simulink model "wavelet_transmux"  (R2018a)
settings: Solver=FixedStepDiscrete  StartTime=0.0  StopTime=inf  RelTol=1e-3
libraries: dspmlti4 x2, dspsrcs4 x1
settings Model: Creator=Kaustubh  LastModifiedBy=Kaustubh
settings SolverCC: AutoInsertRateTranBlk=on
settings DataIOCC: LimitDataPoints=on  SaveOutput=off  SignalLogging=off  SaveTime=off
settings OptimizationCC: LifeSpan=inf  SimCompilerOptimization=on
settings DebuggingCC: AlgebraicLoopMsg=error  SingleTaskRateTransMsg=error  AllowSymbolicDim=off  SFUnexpectedBacktrackingDiag=warning  SFNoUnconditionalDefaultTransitionDiag=warning  SFExecutionAtInitializationDiag=none
settings CodeAppCC: StateflowObjectComments=on
settings GRTTargetCC: TargetLangStandard=C89/C90 (ANSI)  GeneratePreprocessorConditionals=Disable all
settings ConfigComp: CovMetricSettings=dw  CovHtmlReporting=on  CovSaveCumulativeToWorkspaceVar=on  CovSaveSingleToWorkspaceVar=on  CovExternalEMLEnable=off  CovSFcnEnable=off

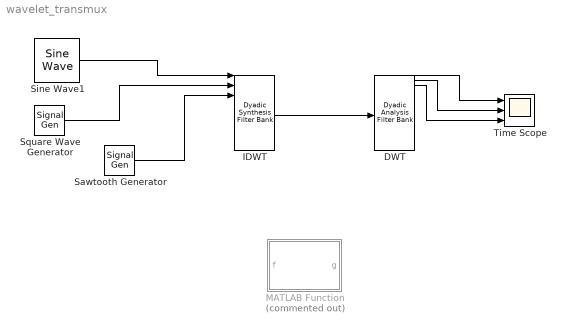
== system wavelet_transmux ==
  DWT : dspmlti4/Dyadic Analysis Filter Bank  Wname=User-defined  OrdRec_ordDec=[1 / 1]  Order=2  LPF=[-0.0105974017849973 0.0328830116669830 0.0308413818359870 -0.187034811718881 -0.0279837694169839 0.630880767929591 0.714846570552542 0.230377813308855]  HPF=[-0.230377813308855 0.714846570552542 -0.630880767929591 -0.0279837694169839 0.187034811718881 0.0308413818359870 -0.0328830116669830 -0.0105974017849973]  NumLevels=4  tree=Symmetric  Output=Multiple ports  OutputFrames=off
      settings: SourceProductName=DSP System Toolbox  SourceProductBaseCode=DS
  IDWT : dspmlti4/Dyadic Synthesis Filter Bank  Wname=User-defined  OrdRec_ordDec=[1 / 1]  Order=2  LPF=[0 0.230377813308855 0.714846570552542 0.630880767929591 -0.0279837694169839 -0.187034811718881 0.0308413818359870 0.0328830116669830 -0.0105974017849973]  HPF=[0 -0.0105974017849973 -0.0328830116669830 0.0308413818359870 0.187034811718881 -0.0279837694169839 -0.630880767929591 0.714846570552542 -0.230377813308855]  NumLevels=4  tree=Symmetric  Input=Multiple ports  OutputFrames=off
      settings: SourceProductName=DSP System Toolbox  SourceProductBaseCode=DS
  MATLAB Function : MATLAB Function  Commented=on  TreatAsAtomicUnit=on
  Sawtooth Generator : SignalGenerator  WaveForm=sawtooth  Units=rad/sec
  Sine Wave1 : dspsrcs4/Sine Wave  Amplitude=1  Frequency=100  Phase=0  SampleMode=Discrete  OutComplex=Real  CompMethod=Trigonometric fcn  TableSize=Speed  SampleTime=1/1000  SamplesPerFrame=1  ResetState=Restart at time zero  OutputFrames=off  dataType=double  wordLen=16  udDataType=sfix(16)  fracBitsMode=Best precision  numFracBits=15  OutDataTypeStr=double  LastOutDataTypeStr=double
  Square Wave Generator : SignalGenerator  WaveForm=square  Units=rad/sec
  Time Scope : Scope  NumInputPorts=3
  wires:
  Sine Wave1/1 -> IDWT/1
  Square Wave Generator/1 -> IDWT/3
  Sawtooth Generator/1 -> IDWT/5
  IDWT/1 -> DWT/1
  DWT/1 -> Time Scope/1
  DWT/2 -> Time Scope/2
  DWT/3 -> Time Scope/3

== matlab function wavelet_transmux/MATLAB Function ==
  data: f input; g output
function g = dwt(f)

h = [-0.230377813308855 0.714846570552542 -0.630880767929591 -0.0279837694169839 0.187034811718881 0.0308413818359870 -0.0328830116669830 -0.0105974017849973];
N = length(h);  
L = length(f);

c = zeros(1,L);
h0 = zeros(1,N);
h1 = zeros(1,N);
d = zeros(1,L);
e = zeros(1,N + 7);

c = f;
h0  = fliplr(h);                          % Scaling filter
h1 = h;  
h1(1:2:N) = -h1(1:2:N);          % Wavelet filter

e = [c(mod((-(N-1):-1),L)+1) c];          % Make periodic

d = conv(e,h1);   d = d(N:2:(N+L-2));     % Convolve & d-sample
e = conv(e,h0);   e = e(N:2:(N+L-2));     % Convolve & d-sample

g = [e,d];                                % The DWT
